simulink model "tras_4_pid"  (Simulink 5.0)
settings: Solver=ode5  StartTime=0.0  StopTime=80  FixedStep=.01  RelTol=1e-3
undefined symbols (not defined in the file): a, b, c, control_a, control_p, d, e, f, force_a, force_p, rpm_a, rpm_p
settings Model: LastModifiedBy=Administrator

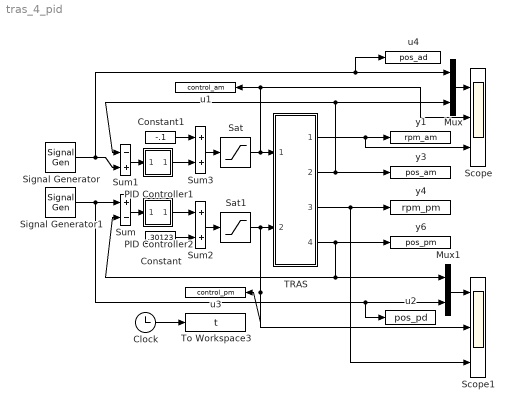
== system tras_4_pid ==
  Clock : Clock
  Constant : Constant  Value=.30123
  Constant1 : Constant  Value=-.1
  Mux : Mux  Inputs=2
  Mux1 : Mux  Inputs=2
  PID Controller1 : Subsystem  AncestorBlock=simulink_extras/Additional Linear/PID Controller  mask(PID Controller){P=a, I=b, D=c, S=1}
      mask prompts: P "Proportional:"; I "Integral:"; D "Derivative:"; S "Integral sat (0-1)"
      mask help:
      | Enter expressions for proportional, integral, and derivative terms.
      | P+I/s+Ds
      mask Help: This block implements a PID controller where parameters are entered for the Proportional, Integral and Derivative terms. Unmask this block to see how it works. The derivative term is implemented using a true derivative block.
      mask Display: disp('PID')
  PID Controller2 : Subsystem  AncestorBlock=simulink_extras/Additional Linear/PID Controller  mask(PID Controller){P=d, I=e, D=f, S=1.4613}
      mask prompts: P "Proportional:"; I "Integral:"; D "Derivative:"; S "Integral sat (0-1)"
      mask help:
      | Enter expressions for proportional, integral, and derivative terms.
      | P+I/s+Ds
      mask Help: This block implements a PID controller where parameters are entered for the Proportional, Integral and Derivative terms. Unmask this block to see how it works. The derivative term is implemented using a true derivative block.
      mask Display: disp('PID')
  Sat : Saturate
  Sat1 : Saturate  UpperLimit=1  LowerLimit=.15
  Scope : Scope  NumInputPorts=3
      settings: YMin=-0.0006~-0.001~0  YMax=0~0.006~40
  Scope1 : Scope  NumInputPorts=3
      settings: YMin=-0.75~-1~-3000  YMax=1.75~1~14000
  Signal Generator : SignalGenerator  WaveForm=square  Amplitude=.1  Frequency=.05
  Signal Generator1 : SignalGenerator  WaveForm=square  Amplitude=.1  Frequency=.025
  Sum : Sum  Inputs=+-  SaturateOnIntegerOverflow=on
  Sum1 : Sum  Inputs=-+  SaturateOnIntegerOverflow=on
  Sum2 : Sum  SaturateOnIntegerOverflow=on
  Sum3 : Sum  SaturateOnIntegerOverflow=on
  TRAS : Subsystem
  To Workspace3 : ToWorkspace  VariableName=t  SampleTime=-1  SaveFormat=Array
  u1 : ToWorkspace  VariableName=control_am  SampleTime=-1  SaveFormat=Array
  u2 : ToWorkspace  VariableName=pos_pd  SampleTime=-1  SaveFormat=Array
  u3 : ToWorkspace  VariableName=control_pm  SampleTime=-1  SaveFormat=Array
  u4 : ToWorkspace  VariableName=pos_ad  SampleTime=-1  SaveFormat=Array
  y1 : ToWorkspace  VariableName=rpm_am  SampleTime=-1  SaveFormat=Array
  y3 : ToWorkspace  VariableName=pos_am  SampleTime=-1  SaveFormat=Array
  y4 : ToWorkspace  VariableName=rpm_pm  SampleTime=-1  SaveFormat=Array
  y6 : ToWorkspace  VariableName=pos_pm  SampleTime=-1  SaveFormat=Array
  wires:
  TRAS/2(pos_a) -> y3/1, Sum1/1, Mux/2
  Clock/1 -> To Workspace3/1
  TRAS/1(rpm_a) -> y1/1, Scope/3
  TRAS/3(rpm_p) -> y4/1, Scope1/3
  TRAS/4(pos_p) -> y6/1, Sum/2, Mux1/1
  Sum/1 -> PID Controller2/1(In_1)
  Sum1/1 -> PID Controller1/1(In_1)
  Sum2/1 -> Sat1/1
  Sat1/1 -> TRAS/2(ctr_p), u3/1, Scope1/2
  Mux/1 -> Scope/1
  Mux1/1 -> Scope1/1
  Signal Generator/1 -> Sum1/2, Mux/1, u4/1
  Signal Generator1/1 -> Sum/1, u2/1, Mux1/2
  Sat/1 -> TRAS/1(ctr_a), u1/1, Scope/2
  Constant/1 -> Sum2/2
  PID Controller2/1(Out_1) -> Sum2/1
  Sum3/1 -> Sat/1
  PID Controller1/1(Out_1) -> Sum3/2
  Constant1/1 -> Sum3/1

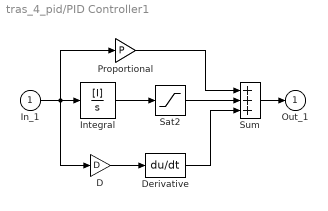
== system tras_4_pid/PID Controller1 ==
  In_1 : Inport
  D : Gain  Gain=D  SaturateOnIntegerOverflow=on
  Derivative : Derivative
  Integral : TransferFcn  Numerator=[I]  Denominator=[1 0]
  Proportional : Gain  Gain=P  SaturateOnIntegerOverflow=on
  Sat2 : Saturate  UpperLimit=S  LowerLimit=-S
  Sum : Sum  Inputs=+++  SaturateOnIntegerOverflow=on  InputSameDT=on
  Out_1 : Outport  InitialOutput=0
  wires:
  Proportional/1 -> Sum/1
  Integral/1 -> Sat2/1
  Derivative/1 -> Sum/3
  In_1/1 -> Integral/1, Proportional/1, D/1
  Sum/1 -> Out_1/1
  D/1 -> Derivative/1
  Sat2/1 -> Sum/2

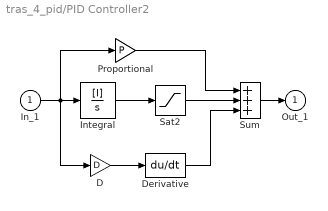
== system tras_4_pid/PID Controller2 ==
  In_1 : Inport
  D : Gain  Gain=D  SaturateOnIntegerOverflow=on
  Derivative : Derivative
  Integral : TransferFcn  Numerator=[I]  Denominator=[1 0]
  Proportional : Gain  Gain=P  SaturateOnIntegerOverflow=on
  Sat2 : Saturate  UpperLimit=S  LowerLimit=-S
  Sum : Sum  Inputs=+++  SaturateOnIntegerOverflow=on  InputSameDT=on
  Out_1 : Outport  InitialOutput=0
  wires:
  Sat2/1 -> Sum/2
  D/1 -> Derivative/1
  Sum/1 -> Out_1/1
  In_1/1 -> D/1, Proportional/1, Integral/1
  Derivative/1 -> Sum/3
  Integral/1 -> Sat2/1
  Proportional/1 -> Sum/1

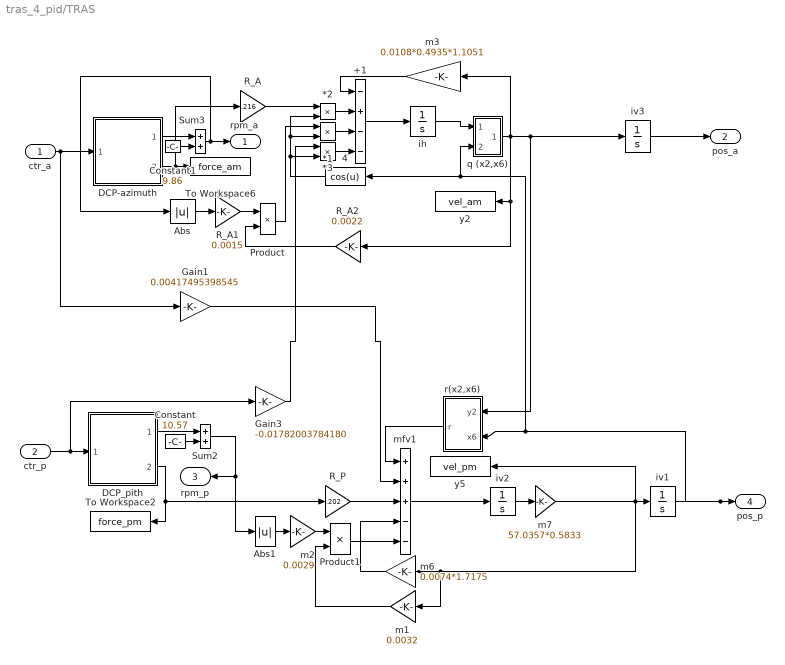
== system tras_4_pid/TRAS ==
  ctr_a : Inport
  ctr_p : Inport  Port=2
  *1 : Product  SaturateOnIntegerOverflow=on  InputSameDT=on
  *2 : Product  SaturateOnIntegerOverflow=on  InputSameDT=on
  *3 : Product  SaturateOnIntegerOverflow=on  InputSameDT=on
  +1 : Sum  Inputs=-+--  SaturateOnIntegerOverflow=on  InputSameDT=on
  4 : Fcn  Orientation=left  Expr=cos(u)
  Abs : Abs  SaturateOnIntegerOverflow=on
  Abs1 : Abs  SaturateOnIntegerOverflow=on
  Constant : Constant  Value=10.57
  Constant1 : Constant  Value=9.86
  DCP-azimuth : Subsystem
  DCP_pith : Subsystem
  Gain1 : Gain  Gain=0.00417495398545  SaturateOnIntegerOverflow=on
  Gain3 : Gain  Gain=-0.01782003784180  SaturateOnIntegerOverflow=on
  Product : Product  SaturateOnIntegerOverflow=on  InputSameDT=on
  Product1 : Product  SaturateOnIntegerOverflow=on
  R_A : Gain  Gain=.216
  R_A1 : Gain  Gain=0.0015
  R_A2 : Gain  Orientation=left  Gain=0.0022
  R_P : Gain  Gain=.202
  Sum2 : Sum  SaturateOnIntegerOverflow=on
  Sum3 : Sum  SaturateOnIntegerOverflow=on
  To Workspace2 : ToWorkspace  VariableName=force_pm  SampleTime=-1  SaveFormat=Array
  To Workspace6 : ToWorkspace  VariableName=force_am  SampleTime=-1  SaveFormat=Array
  ih : Integrator  LimitOutput=on  UpperSaturationLimit=10  LowerSaturationLimit=-10
  iv1 : Integrator  InitialCondition=-.5319*0  UpperSaturationLimit=pi  LowerSaturationLimit=-pi
  iv2 : Integrator  UpperSaturationLimit=pi  LowerSaturationLimit=-pi
  iv3 : Integrator  LimitOutput=on  UpperSaturationLimit=6  LowerSaturationLimit=-6
  m1 : Gain  Orientation=left  Gain=0.0032  SaturateOnIntegerOverflow=on
  m2 : Gain  Gain=0.0029  SaturateOnIntegerOverflow=on
  m3 : Gain  Orientation=left  Gain=0.0108*0.4935*1.1051
  m6 : Gain  Orientation=left  Gain=0.0074*1.7175
  m7 : Gain  Gain=57.0357*0.5833  SaturateOnIntegerOverflow=on
  mfv1 : Sum  Inputs=+++--  SaturateOnIntegerOverflow=on  InputSameDT=on
  q (x2,x6) : Subsystem
  r(x2,x6) : Subsystem  Orientation=left
  y2 : ToWorkspace  VariableName=vel_am  SampleTime=-1  SaveFormat=Array
  y5 : ToWorkspace  VariableName=vel_pm  SampleTime=-1  SaveFormat=Array
  rpm_a : Outport
  pos_a : Outport  Port=2
  rpm_p : Outport  Orientation=left  Port=3
  pos_p : Outport  Port=4
  wires:
  DCP-azimuth/2(FORCE_A) -> To Workspace6/1, R_A/1
  DCP-azimuth/1(RPM_A) -> Sum3/1
  *1/1 -> +1/3
  m3/1 -> +1/1
  *2/1 -> +1/2
  ih/1 -> q (x2,x6)/1(x2)
  q (x2,x6)/1(q) -> R_A2/1, y2/1, iv3/1, r(x2,x6)/1(y2), m3/1
  R_A/1 -> *2/1
  Abs/1 -> R_A1/1
  R_A1/1 -> Product/1
  R_A2/1 -> Product/2
  DCP_pith/2(FORCE_P) -> To Workspace2/1, R_P/1
  m6/1 -> mfv1/4
  iv2/1 -> m7/1
  mfv1/1 -> iv2/1
  m7/1 -> y5/1, iv1/1, m6/1, m1/1
  DCP_pith/1(RPM_P) -> Sum2/1
  Abs1/1 -> m2/1
  Product1/1 -> mfv1/5
  r(x2,x6)/1(r) -> mfv1/1
  R_P/1 -> mfv1/3
  iv1/1 -> 4/1, q (x2,x6)/2(x6), r(x2,x6)/2(x6), pos_p/1
  m1/1 -> Product1/2
  m2/1 -> Product1/1
  *3/1 -> +1/4
  Product/1 -> *1/1
  4/1 -> *2/2, *1/2, *3/2
  Gain1/1 -> mfv1/2
  Gain3/1 -> *3/1
  ctr_a/1 -> Gain1/1, DCP-azimuth/1(CTR_A)
  ctr_p/1 -> DCP_pith/1(CTR_P), Gain3/1
  iv3/1 -> pos_a/1
  +1/1 -> ih/1
  Sum2/1 -> Abs1/1, rpm_p/1
  Constant/1 -> Sum2/2
  Sum3/1 -> rpm_a/1, Abs/1
  Constant1/1 -> Sum3/2

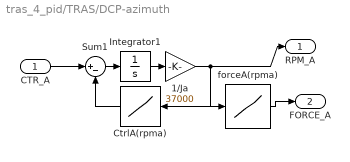
== system tras_4_pid/TRAS/DCP-azimuth ==
  CTR_A : Inport
  1/Ja : Gain  Gain=37000  ShowAdditionalParam=on  SaturateOnIntegerOverflow=on
  CtrlA(rpma) : Lookup  Orientation=left  InputValues=rpm_a  OutputValues=control_a  SaturateOnIntegerOverflow=on
  Integrator1 : Integrator
  Sum1 : Sum  Inputs=|+-  SaturateOnIntegerOverflow=on  InputSameDT=on
  forceA(rpma) : Lookup  InputValues=rpm_a  OutputValues=force_a  SaturateOnIntegerOverflow=on
  RPM_A : Outport
  FORCE_A : Outport  Port=2
  wires:
  Sum1/1 -> Integrator1/1
  CtrlA(rpma)/1 -> Sum1/2
  Integrator1/1 -> 1/Ja/1
  1/Ja/1 -> CtrlA(rpma)/1, forceA(rpma)/1, RPM_A/1
  CTR_A/1 -> Sum1/1
  forceA(rpma)/1 -> FORCE_A/1

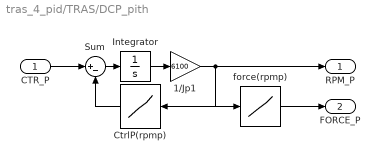
== system tras_4_pid/TRAS/DCP_pith ==
  CTR_P : Inport
  1/Jp1 : Gain  Gain=6100  ShowAdditionalParam=on
  CtrlP(rpmp) : Lookup  Orientation=left  InputValues=rpm_p  OutputValues=control_p  SaturateOnIntegerOverflow=on
  Integrator : Integrator
  Sum : Sum  Inputs=|+-  SaturateOnIntegerOverflow=on  InputSameDT=on
  force(rpmp) : Lookup  InputValues=rpm_p  OutputValues=force_p  SaturateOnIntegerOverflow=on
  RPM_P : Outport
  FORCE_P : Outport  Port=2
  wires:
  Sum/1 -> Integrator/1
  Integrator/1 -> 1/Jp1/1
  CtrlP(rpmp)/1 -> Sum/2
  1/Jp1/1 -> CtrlP(rpmp)/1, force(rpmp)/1, RPM_P/1
  CTR_P/1 -> Sum/1
  force(rpmp)/1 -> FORCE_P/1

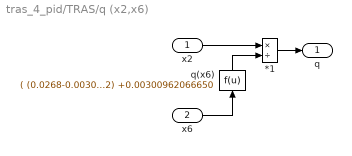
== system tras_4_pid/TRAS/q (x2,x6) ==
  x2 : Inport
  x6 : Inport  Port=2
  " q(x6)" : Fcn  Orientation=up  Expr=( (0.0268-0.00300962066650)*cos(u)^2) +0.00300962066650
  *1 : Product  Inputs=*/  SaturateOnIntegerOverflow=on  InputSameDT=on
  q : Outport
  wires:
  *1/1 -> q/1
  x2/1 -> *1/1
  x6/1 -> " q(x6)"/1
  " q(x6)"/1 -> *1/2

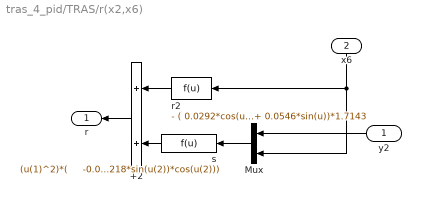
== system tras_4_pid/TRAS/r(x2,x6) ==
  y2 : Inport  Orientation=left
  x6 : Inport  Orientation=down  Port=2
  +2 : Sum  Orientation=left  SaturateOnIntegerOverflow=on  InputSameDT=on
  Mux : Mux  Orientation=left  Inputs=2
  r2 : Fcn  Orientation=left  Expr=- ( 0.0292*cos(u)+ 0.0546*sin(u))*1.7143
  s : Fcn  Orientation=left  Expr="(u(1)^2)*(     -0.07389953104162*  0.28753198180218*sin(u(2))*cos(u(2)))"
  r : Outport  Orientation=left
  wires:
  Mux/1 -> s/1
  r2/1 -> +2/1
  s/1 -> +2/2
  x6/1 -> Mux/2, r2/1
  +2/1 -> r/1
  y2/1 -> Mux/1
